simulink model "Model"  (R2018a)
settings: Solver=VariableStepAuto  StartTime=0.0  StopTime=1000  FixedStep=1/480  RelTol=1e-2  EnableMultiTasking=on
model workspace (MAT data in the model file):
  t = Simulink.Parameter
  t.DataType = 'auto'
  t.Dimensions = [0 0]
undefined symbols (not defined in the file or in its folder): deg, Earth, F, Light, MIL, rad, Receive, s, Send, WGS84
libraries: simulink_extras x7, aerolibfltsims x4, aerolibconvert2 x4, aerolibwind2 x3, aerolibtransform2 x1, aerolibatmos2 x1, sharedtransform x1, aerolibanimutils x1, aerolibasang x1
settings Model: Creator=venge  LastModifiedBy=venge
settings SolverCC: AlgebraicLoopSolver=LineSearch  AutoInsertRateTranBlk=on
settings OptimizationCC: LifeSpan=inf
settings DebuggingCC: MaxConsecutiveZCsMsg=warning  ModelReferenceExtraNoncontSigs=warning  SFUnexpectedBacktrackingDiag=warning  SFNoUnconditionalDefaultTransitionDiag=warning  SFExecutionAtInitializationDiag=none
settings CodeAppCC: StateflowObjectComments=on
settings GRTTargetCC: TargetLangStandard=C89/C90 (ANSI)  GeneratePreprocessorConditionals=Disable all
settings ConfigComp: CovMetricSettings=dw  CovHtmlReporting=on  CovSaveCumulativeToWorkspaceVar=on  CovSaveSingleToWorkspaceVar=on  CovExternalEMLEnable=off

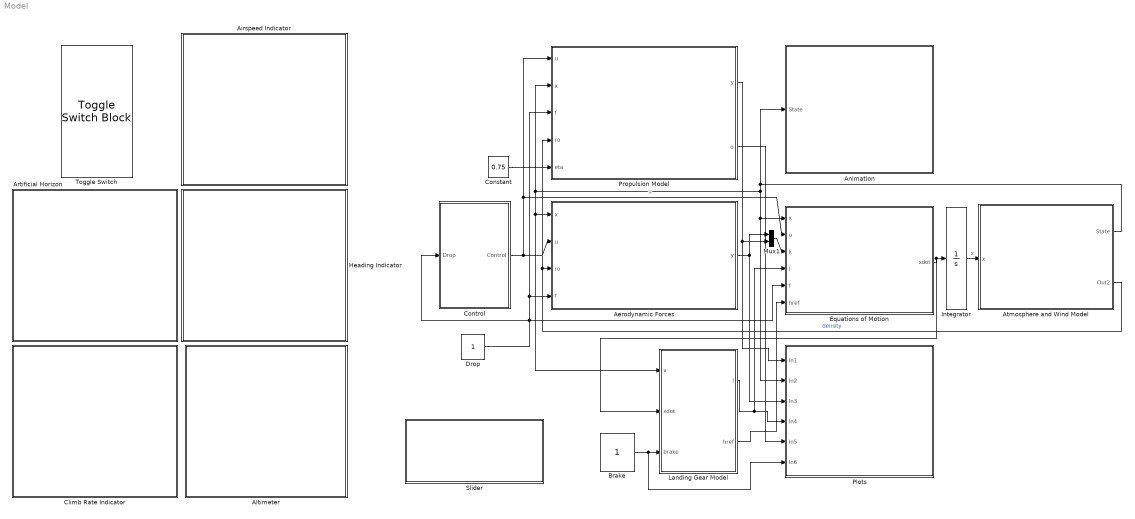
== system Model ==
  "Aerodynamic Forces " : MATLAB Function  TreatAsAtomicUnit=on
  Airspeed Indicator : Subsystem  DialogController=aeroblksHMICreateDDGDialog  IsWebBlock=on  mask(MWDashboardBlock){webBlockId=31f690db-bb0a-4ac4-9dff-202d3d07e85e, webBlockType=airspeedindicator, ShowInLibBrowser=on, ShowInitialText=on, HMISrcModelName=Model}
      mask prompts: webBlockId "WebBlock Id"; webBlockType "WebBlock Type"; HMISrcModelName "Source Model"
      mask help: aeroblksHMI:aeroblkhmi:AirspeedIndicatorDialogDesc
      mask Help: eval('asbhmihelp(''airspeedindicator'')');
      mask Display:
      | if strcmp(get_param(bdroot(gcb),'BlockDiagramType'), 'library')
      |  image([(matlabroot) '/toolbox/aeroblks/aeroblks/hmi/icons/AirspeedIndicatorIcon.svg'])
      | end
  Altimeter : Subsystem  DialogController=aeroblksHMICreateDDGDialog  IsWebBlock=on  mask(MWDashboardBlock){webBlockId=98444758-a21f-440e-aafb-46ae4afdabfa, webBlockType=altimeter, ShowInLibBrowser=on, ShowInitialText=on, HMISrcModelName=Model}
      mask prompts: webBlockId "WebBlock Id"; webBlockType "WebBlock Type"; HMISrcModelName "Source Model"
      mask help: aeroblksHMI:aeroblkhmi:AltimeterDialogDesc
      mask Help: eval('asbhmihelp(''altimeter'')');
      mask Display:
      | if strcmp(get_param(bdroot(gcb),'BlockDiagramType'), 'library')
      |  image([(matlabroot) '/toolbox/aeroblks/aeroblks/hmi/icons/AltimeterIcon.svg'])
      | end
  Animation : Subsystem
      mask Display: image('C:\Users\venge\Documents\Thesis\Flight_Simulator\assets\Animation.png');
  Artificial Horizon : Subsystem  DialogController=aeroblksHMICreateDDGDialog  IsWebBlock=on  mask(MWDashboardBlock){webBlockId=0a6384c6-9f4b-45f8-990f-726f75900e1f, webBlockType=artificialhorizon, ShowInLibBrowser=on, ShowInitialText=on, HMISrcModelName=Model}
      mask prompts: webBlockId "WebBlock Id"; webBlockType "WebBlock Type"; HMISrcModelName "Source Model"
      mask help: aeroblksHMI:aeroblkhmi:ArtificialHorizonDialogDesc
      mask Help: eval('asbhmihelp(''artificialhorizon'')');
      mask Display:
      | if strcmp(get_param(bdroot(gcb),'BlockDiagramType'), 'library')
      |  image([(matlabroot) '/toolbox/aeroblks/aeroblks/hmi/icons/ArtificialHorizonIcon.svg'])
      | end
  Atmosphere and Wind Model : Subsystem
      mask Display: image('C:\Users\venge\Documents\Thesis\Flight_Simulator\assets\Wind.jpg');
  Climb Rate Indicator : Subsystem  DialogController=aeroblksHMICreateDDGDialog  IsWebBlock=on  mask(MWDashboardBlock){webBlockId=41f67cdb-ffed-4f88-bf4d-534dd7e67a65, webBlockType=climbindicator, ShowInLibBrowser=on, ShowInitialText=on, HMISrcModelName=Model}
      mask prompts: webBlockId "WebBlock Id"; webBlockType "WebBlock Type"; HMISrcModelName "Source Model"
      mask help: aeroblksHMI:aeroblkhmi:ClimbIndicatorDialogDesc
      mask Help: eval('asbhmihelp(''climbindicator'')');
      mask Display:
      | if strcmp(get_param(bdroot(gcb),'BlockDiagramType'), 'library')
      |  image([(matlabroot) '/toolbox/aeroblks/aeroblks/hmi/icons/ClimbIndicatorIcon.svg'])
      | end
  Constant : Constant  Value=0.75
  Control : Subsystem
      mask Display: image('C:\Users\venge\Documents\Thesis\Flight_Simulator\assets\Joystick.jpg');
  Drop : Constant
  "Equations of Motion " : MATLAB Function  TreatAsAtomicUnit=on
  Heading Indicator : Subsystem  DialogController=aeroblksHMICreateDDGDialog  IsWebBlock=on  mask(MWDashboardBlock){webBlockId=bb5b7226-34b9-44e0-9042-3ee55364d958, webBlockType=headingindicator, ShowInLibBrowser=on, ShowInitialText=on, HMISrcModelName=Model}
      mask prompts: webBlockId "WebBlock Id"; webBlockType "WebBlock Type"; HMISrcModelName "Source Model"
      mask help: aeroblksHMI:aeroblkhmi:HeadingIndicatorDialogDesc
      mask Help: eval('asbhmihelp(''headingindicator'')');
      mask Display:
      | if strcmp(get_param(bdroot(gcb),'BlockDiagramType'), 'library')
      |  image([(matlabroot) '/toolbox/aeroblks/aeroblks/hmi/icons/HeadingIndicatorIcon.svg'])
      | end
  Integrator : Integrator  InitialCondition=[30 0 0 0 0 0 0 0 0 0 0 -50]'
  Landing Gear Model : Subsystem
      mask Display: image('C:\Users\venge\Documents\Thesis\Flight_Simulator\assets\LandingGear.jpeg');
  Mux1 : Mux  Inputs=2
  Plots : Subsystem
      mask Display: image('C:\Users\venge\Documents\Thesis\Flight_Simulator\assets\Graph.jpg');
  Propulsion Model : MATLAB Function  TreatAsAtomicUnit=on
  Slider : Subsystem  DialogController=hmiCreateDDGDialog  IsWebBlock=on  mask(MWDashboardBlock){webBlockId=e69ca618-8fcc-4738-b870-e52728e9a647, webBlockType=slider, ShowInLibBrowser=on, ShowInitialText=on, HMISrcModelName=Model}
      mask prompts: webBlockId "WebBlock Id"; webBlockType "WebBlock Type"; HMISrcModelName "Source Model"
      mask help: SimulinkHMI:dialogs:SliderDialogDesc
      mask Help: helpview([docroot '/mapfiles/simulink.map'], 'hmi_slider')
      mask Display:
      | if strcmp(get_param(bdroot(gcb),'BlockDiagramType'), 'library')
      |     image([(matlabroot) '/toolbox/simulink/hmi/icons/Slider.png']);
      | end
  Toggle Switch : ToggleSwitchBlock  WebBlockId=379  LabelPosition=Hide
      settings: Values={{'Off', 'On'}, [0 1]}
  Βrake : Constant
  wires:
  Control/1(Control) -> "Equations of Motion "/2(u), Propulsion Model/1(u), "Aerodynamic Forces "/2(u)  "u"
  "Aerodynamic Forces "/1(y) -> Mux1/1, Plots/3(In3)
  Propulsion Model/1(y) -> Plots/1(In1), Mux1/2
  Mux1/1 -> "Equations of Motion "/3(k)
  Atmosphere and Wind Model/1(State) -> Plots/2(In2), "Equations of Motion "/1(x), Propulsion Model/2(x), Landing Gear Model/1(x), "Aerodynamic Forces "/1(x), Animation/1(State)
  Integrator/1 -> Atmosphere and Wind Model/1(x)  "x"
  Landing Gear Model/1(l) -> Plots/4(In4), "Equations of Motion "/4(l)
  Βrake/1 -> Plots/6(In6), Landing Gear Model/3(brake)
  Atmosphere and Wind Model/2(Out2) -> Propulsion Model/4(ro), "Aerodynamic Forces "/3(ro)  "density"
  "Equations of Motion "/1(xdot) -> Landing Gear Model/2(xdot), Integrator/1
  Drop/1 -> Control/1(Drop), Propulsion Model/3(f), "Aerodynamic Forces "/4(f), "Equations of Motion "/5(f)
  Propulsion Model/2(o) -> Plots/5(In5)
  Constant/1 -> Propulsion Model/5(eta)
  Landing Gear Model/2(href) -> "Equations of Motion "/6(href)

== system Model/Airspeed Indicator ==

== system Model/Altimeter ==

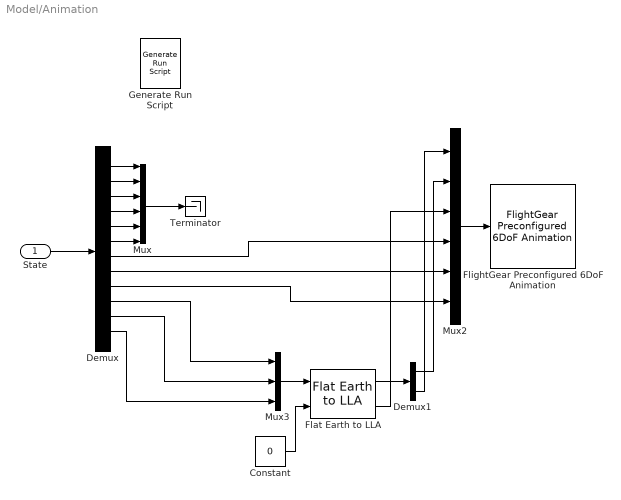
== system Model/Animation ==
  State : Inport
  Constant : Constant  Value=0
  Demux : Demux  Outputs=12
  Demux1 : Demux  Outputs=2
  Flat Earth to LLA : aerolibtransform2/Flat Earth to LLA  units=Metric (MKS)  ptype=Earth (WGS84)  F=1/298.257223563  R=6378137  LL0=[37.6069 -122.381]  psi=0
  FlightGear Preconfigured 6DoF Animation : aerolibfltsims/FlightGear Preconfigured 6DoF Animation  xFlightGearVersion=v2017.3  DestinationIpAddress=127.0.0.1  DestinationPort=5502  SampleTime=1/30
      settings: SourceProductName=Aerospace Blockset
  Generate Run Script : aerolibfltsims/Generate Run Script  Architecture=Default  dataFlow=Send-Receive  GeometryModelName=c172p  AirportId=KSFO  RunwayId=10L  InitialAltitude=2000  InitialHeading=0  OffsetDistance=0  OffsetAzimuth=0  InstallScenery=on  DisableShaders=on  OriginAddress=127.0.0.1  DestinationPort=5502  OriginPort=5505  LocalAddress=127.0.0.1  OutputFileName=runfg_send_recieve.bat  FlightGearBaseDirectory=C:\Program Files\FlightGear 2017.3.1
  Mux : Mux  Inputs=6
  Mux2 : Mux  Inputs=6
  Mux3 : Mux  Inputs=3
  Terminator : Terminator
  wires:
  Demux1/2 -> Mux2/1
  Flat Earth to LLA/1 -> Demux1/1
  Demux1/1 -> Mux2/2
  Mux2/1 -> FlightGear Preconfigured 6DoF Animation/1
  Flat Earth to LLA/2 -> Mux2/3
  Mux3/1 -> Flat Earth to LLA/1
  State/1 -> Demux/1
  Demux/10 -> Mux3/1
  Demux/11 -> Mux3/2
  Demux/12 -> Mux3/3
  Demux/7 -> Mux2/4
  Demux/9 -> Mux2/6
  Demux/6 -> Mux/6
  Demux/5 -> Mux/5
  Demux/4 -> Mux/4
  Demux/3 -> Mux/3
  Demux/2 -> Mux/2
  Demux/1 -> Mux/1
  Mux/1 -> Terminator/1
  Demux/8 -> Mux2/5
  Constant/1 -> Flat Earth to LLA/2

== system Model/Artificial Horizon ==

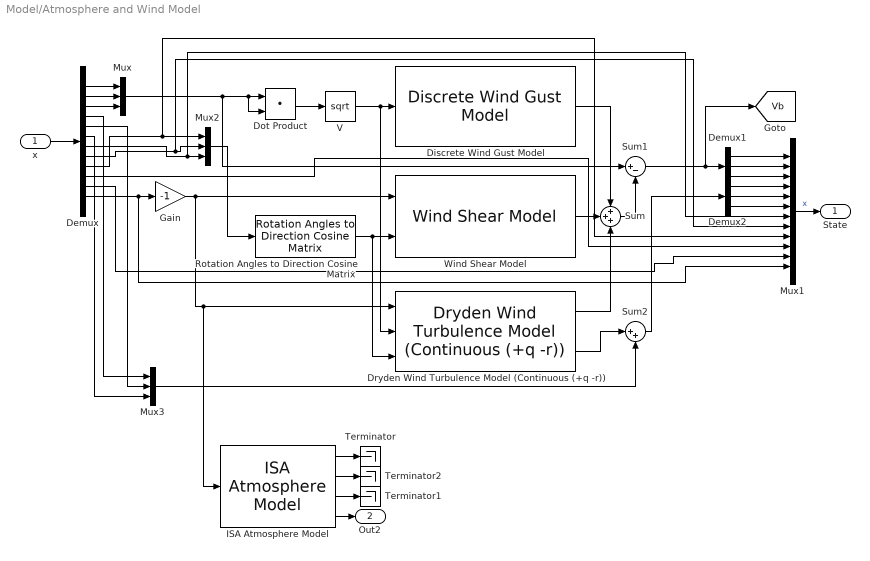
== system Model/Atmosphere and Wind Model ==
  x : Inport
  Demux : Demux  Outputs=12
  Demux1 : Demux  Outputs=3
  Demux2 : Demux  Outputs=3
  Discrete Wind Gust Model : aerolibwind2/Discrete Wind Gust Model  units=Metric (MKS)  Gx=off  Gy=off  Gz=off  t_0=50  d_m=[200 200 200]  v_m=[20 -20 20]
      settings: SourceProductName=Aerospace Blockset
  Dot Product : DotProduct  InputSameDT=on  OutDataTypeStr=Inherit: Inherit via internal rule
  Dryden Wind Turbulence Model (Continuous (+q -r)) : aerolibwind2/Dryden Wind Turbulence Model  (Continuous (+q -r))  units=Metric (MKS)  spec=MIL-F-8785C  model=Continuous Dryden (-q +r)  W20=0  Wdeg=0  TurbProb=10^-2 - Light  L_high=533.4  Wingspan=7.146  ts=0.1  Seed=[23341 23342 23343 23344]  T_on=off
      settings: SourceProductName=Aerospace Blockset
  Gain : Gain  Gain=-1
  ISA Atmosphere Model : aerolibatmos2/ISA Atmosphere Model  custom=off  g=9.80665  gamma=1.4  R=287.0531  L=0.0065  h_trop=11000  h_strat=20000  rho0=1.225  P0=101325  T0=288.15  h0=0
      settings: SourceProductName=Aerospace Blockset
  Mux : Mux  Inputs=3
  Mux1 : Mux  Inputs=12
  Mux2 : Mux  Inputs=3
  Mux3 : Mux  Inputs=3
  Rotation Angles to Direction Cosine Matrix : sharedtransform/Rotation Angles to Direction Cosine Matrix  rotationOrder=ZYX  aMode=aMode
      settings: SourceProductBaseCode=AE
  Sum : Sum  Inputs=+++
  Sum1 : Sum  Inputs=|+-
  Sum2 : Sum  Inputs=|++
  Terminator : Terminator
  Terminator1 : Terminator
  Terminator2 : Terminator
  V : Sqrt  SaturateOnIntegerOverflow=on
  Wind Shear Model : aerolibwind2/Wind Shear Model  units=Metric (MKS)  phase=Other  W_20=0  Wdeg=0
      settings: SourceProductName=Aerospace Blockset
  State : Outport  PortDimensions=12
  Out2 : Outport  Port=2
  tag scope: Vb=global
  wires:
  Demux/2 -> Mux/2
  Demux/3 -> Mux/3
  Demux/1 -> Mux/1
  Sum2/1 -> Demux2/1
  Mux3/1 -> Sum2/2
  Mux/1 -> Sum1/1, Dot Product/2, Dot Product/1
  Mux2/1 -> Rotation Angles to Direction Cosine Matrix/1
  Gain/1 -> ISA Atmosphere Model/1, Dryden Wind Turbulence Model (Continuous (+q -r))/1, Wind Shear Model/1
  Demux/12 -> Mux1/12, Gain/1
  Discrete Wind Gust Model/1 -> Sum/1
  Sum/1 -> Sum1/2
  V/1 -> Dryden Wind Turbulence Model (Continuous (+q -r))/2, Discrete Wind Gust Model/1
  Rotation Angles to Direction Cosine Matrix/1 -> Dryden Wind Turbulence Model (Continuous (+q -r))/3, Wind Shear Model/2
  Dryden Wind Turbulence Model (Continuous (+q -r))/1 -> Sum/3
  Dot Product/1 -> V/1
  Wind Shear Model/1 -> Sum/2
  Dryden Wind Turbulence Model (Continuous (+q -r))/2 -> Sum2/1
  Mux1/1 -> State/1  "x"
  x/1 -> Demux/1
  Demux1/1 -> Mux1/1
  Demux1/2 -> Mux1/2
  Demux1/3 -> Mux1/3
  Demux/4 -> Mux3/1
  Demux/5 -> Mux3/2
  Demux/6 -> Mux3/3
  Demux/7 -> Mux1/7, Mux2/3
  Demux/8 -> Mux1/8, Mux2/2
  Demux/9 -> Mux1/9, Mux2/1
  Demux/10 -> Mux1/10
  Demux/11 -> Mux1/11
  Demux2/1 -> Mux1/4
  Demux2/2 -> Mux1/5
  Demux2/3 -> Mux1/6
  ISA Atmosphere Model/3 -> Terminator1/1
  ISA Atmosphere Model/1 -> Terminator/1
  ISA Atmosphere Model/2 -> Terminator2/1
  ISA Atmosphere Model/4 -> Out2/1
  Sum1/1 -> [Vb], Demux1/1

== system Model/Climb Rate Indicator ==

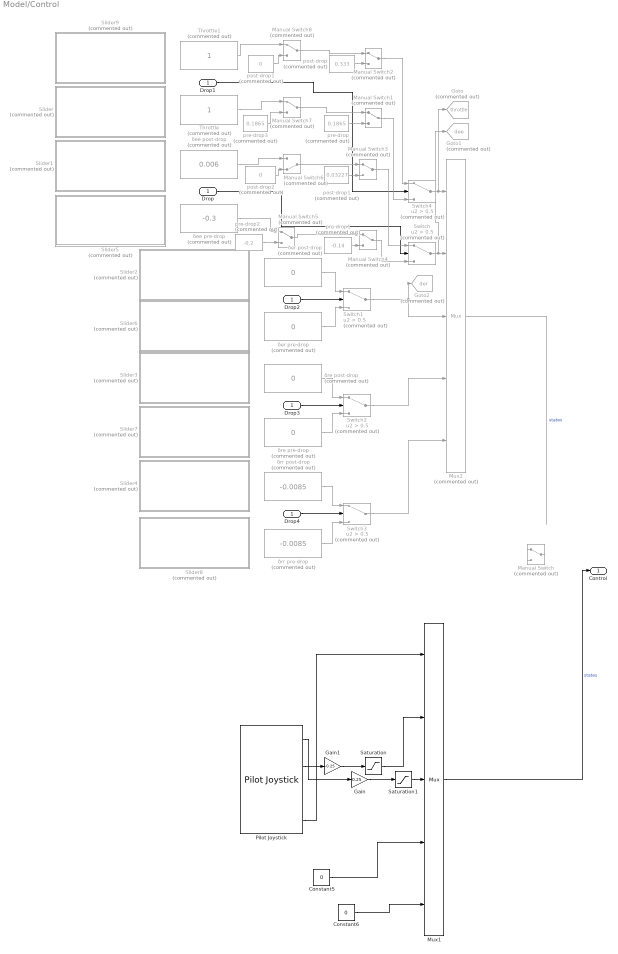
== system Model/Control ==
  Drop : Inport
  Constant5 : Constant  Value=0
  Constant6 : Constant  Value=0
  Drop{1..4} (4 alike) : InportShadow
  Gain : Gain  Gain=0.25
  Gain1 : Gain  Gain=-0.25
  Goto : Goto  Commented=on  GotoTag=throttle  TagVisibility=global
  Goto1 : Goto  Commented=on  GotoTag=dee  TagVisibility=global
  Goto2 : Goto  Commented=on  GotoTag=der  TagVisibility=global
  Manual Switch{,1..5,7..8} (8 alike) : ManualSwitch  Commented=on
  Manual Switch6 : ManualSwitch  Commented=on  CurrentSetting=0
  Mux1 : Mux  Inputs=5
  Mux2 : Mux  Commented=on  Inputs=5
  Pilot Joystick : aerolibanimutils/Pilot Joystick  JoystickID=Joystick1  OutputConfiguration=FourAxis  SampleTime=1/30
  Saturation : Saturate  UpperLimit=0.4  LowerLimit=-0.4
  Saturation1 : Saturate  UpperLimit=0.4  LowerLimit=-0.4
  Slider : Subsystem  Commented=on  DialogController=hmiCreateDDGDialog  IsWebBlock=on  mask(MWDashboardBlock){webBlockId=71ff8332-cc57-48c6-a6db-909c0a3f45d7, webBlockType=slider, ShowInLibBrowser=on, ShowInitialText=on, HMISrcModelName=Model}
      mask prompts: webBlockId "WebBlock Id"; webBlockType "WebBlock Type"; HMISrcModelName "Source Model"
      mask Help: helpview([docroot '/mapfiles/simulink.map'], 'hmi_slider')
      mask Display:
      | if strcmp(get_param(bdroot(gcb),'BlockDiagramType'), 'library')
      |     image([(matlabroot) '/toolbox/simulink/hmi/icons/Slider.png']);
      | end
  Slider1 : Subsystem  Commented=on  DialogController=hmiCreateDDGDialog  IsWebBlock=on  mask(MWDashboardBlock){webBlockId=76778588-3397-48c9-bd33-f2999619dd82, webBlockType=slider, ShowInLibBrowser=on, ShowInitialText=on, HMISrcModelName=Model}
      mask prompts: webBlockId "WebBlock Id"; webBlockType "WebBlock Type"; HMISrcModelName "Source Model"
      mask Help: helpview([docroot '/mapfiles/simulink.map'], 'hmi_slider')
      mask Display:
      | if strcmp(get_param(bdroot(gcb),'BlockDiagramType'), 'library')
      |     image([(matlabroot) '/toolbox/simulink/hmi/icons/Slider.png']);
      | end
  Slider2 : Subsystem  Commented=on  DialogController=hmiCreateDDGDialog  IsWebBlock=on  mask(MWDashboardBlock){webBlockId=50b965dc-06ed-4b8f-b83d-27d9610c145d, webBlockType=slider, ShowInLibBrowser=on, ShowInitialText=on, HMISrcModelName=Model}
      mask prompts: webBlockId "WebBlock Id"; webBlockType "WebBlock Type"; HMISrcModelName "Source Model"
      mask Help: helpview([docroot '/mapfiles/simulink.map'], 'hmi_slider')
      mask Display:
      | if strcmp(get_param(bdroot(gcb),'BlockDiagramType'), 'library')
      |     image([(matlabroot) '/toolbox/simulink/hmi/icons/Slider.png']);
      | end
  Slider3 : Subsystem  Commented=on  DialogController=hmiCreateDDGDialog  IsWebBlock=on  mask(MWDashboardBlock){webBlockId=b80eeb05-1d01-4bba-9885-77def870bdbb, webBlockType=slider, ShowInLibBrowser=on, ShowInitialText=on, HMISrcModelName=Model}
      mask prompts: webBlockId "WebBlock Id"; webBlockType "WebBlock Type"; HMISrcModelName "Source Model"
      mask Help: helpview([docroot '/mapfiles/simulink.map'], 'hmi_slider')
      mask Display:
      | if strcmp(get_param(bdroot(gcb),'BlockDiagramType'), 'library')
      |     image([(matlabroot) '/toolbox/simulink/hmi/icons/Slider.png']);
      | end
  Slider4 : Subsystem  Commented=on  DialogController=hmiCreateDDGDialog  IsWebBlock=on  mask(MWDashboardBlock){webBlockId=fbe885e3-15c5-4246-8884-16500feaa139, webBlockType=slider, ShowInLibBrowser=on, ShowInitialText=on, HMISrcModelName=Model}
      mask prompts: webBlockId "WebBlock Id"; webBlockType "WebBlock Type"; HMISrcModelName "Source Model"
      mask Help: helpview([docroot '/mapfiles/simulink.map'], 'hmi_slider')
      mask Display:
      | if strcmp(get_param(bdroot(gcb),'BlockDiagramType'), 'library')
      |     image([(matlabroot) '/toolbox/simulink/hmi/icons/Slider.png']);
      | end
  Slider5 : Subsystem  Commented=on  DialogController=hmiCreateDDGDialog  IsWebBlock=on  mask(MWDashboardBlock){webBlockId=8ae96144-d421-4708-bdd7-b0b2312d1c18, webBlockType=slider, ShowInLibBrowser=on, ShowInitialText=on, HMISrcModelName=Model}
      mask prompts: webBlockId "WebBlock Id"; webBlockType "WebBlock Type"; HMISrcModelName "Source Model"
      mask Help: helpview([docroot '/mapfiles/simulink.map'], 'hmi_slider')
      mask Display:
      | if strcmp(get_param(bdroot(gcb),'BlockDiagramType'), 'library')
      |     image([(matlabroot) '/toolbox/simulink/hmi/icons/Slider.png']);
      | end
  Slider6 : Subsystem  Commented=on  DialogController=hmiCreateDDGDialog  IsWebBlock=on  mask(MWDashboardBlock){webBlockId=9b86d56f-dae5-440b-8eb5-941c5f267d11, webBlockType=slider, ShowInLibBrowser=on, ShowInitialText=on, HMISrcModelName=Model}
      mask prompts: webBlockId "WebBlock Id"; webBlockType "WebBlock Type"; HMISrcModelName "Source Model"
      mask Help: helpview([docroot '/mapfiles/simulink.map'], 'hmi_slider')
      mask Display:
      | if strcmp(get_param(bdroot(gcb),'BlockDiagramType'), 'library')
      |     image([(matlabroot) '/toolbox/simulink/hmi/icons/Slider.png']);
      | end
  Slider7 : Subsystem  Commented=on  DialogController=hmiCreateDDGDialog  IsWebBlock=on  mask(MWDashboardBlock){webBlockId=463fa428-adca-439c-b2e0-0a9da63c573c, webBlockType=slider, ShowInLibBrowser=on, ShowInitialText=on, HMISrcModelName=Model}
      mask prompts: webBlockId "WebBlock Id"; webBlockType "WebBlock Type"; HMISrcModelName "Source Model"
      mask Help: helpview([docroot '/mapfiles/simulink.map'], 'hmi_slider')
      mask Display:
      | if strcmp(get_param(bdroot(gcb),'BlockDiagramType'), 'library')
      |     image([(matlabroot) '/toolbox/simulink/hmi/icons/Slider.png']);
      | end
  Slider8 : Subsystem  Commented=on  DialogController=hmiCreateDDGDialog  IsWebBlock=on  mask(MWDashboardBlock){webBlockId=151de3c8-e2fa-4a35-b614-725181a5af33, webBlockType=slider, ShowInLibBrowser=on, ShowInitialText=on, HMISrcModelName=Model}
      mask prompts: webBlockId "WebBlock Id"; webBlockType "WebBlock Type"; HMISrcModelName "Source Model"
      mask Help: helpview([docroot '/mapfiles/simulink.map'], 'hmi_slider')
      mask Display:
      | if strcmp(get_param(bdroot(gcb),'BlockDiagramType'), 'library')
      |     image([(matlabroot) '/toolbox/simulink/hmi/icons/Slider.png']);
      | end
  Slider9 : Subsystem  Commented=on  DialogController=hmiCreateDDGDialog  IsWebBlock=on  mask(MWDashboardBlock){webBlockId=f535e40a-6bfd-4d60-87e7-b92c922fa0f7, webBlockType=slider, ShowInLibBrowser=on, ShowInitialText=on, HMISrcModelName=Model}
      mask prompts: webBlockId "WebBlock Id"; webBlockType "WebBlock Type"; HMISrcModelName "Source Model"
      mask Help: helpview([docroot '/mapfiles/simulink.map'], 'hmi_slider')
      mask Display:
      | if strcmp(get_param(bdroot(gcb),'BlockDiagramType'), 'library')
      |     image([(matlabroot) '/toolbox/simulink/hmi/icons/Slider.png']);
      | end
  Switch{,1..4} (5 alike) : Switch  Commented=on  Criteria=u2 > Threshold  Threshold=0.5
  Throttle : Constant  Commented=on
  Throttle1 : Constant  Commented=on
  post-drop1 : Constant  Commented=on  Value=0.03227
  post-drop2 : Constant  Commented=on  Value=0
  pre-drop : Constant  Commented=on  Value=0.1865
  pre-drop1 : Constant  Commented=on  Value=-0.14
  pre-drop2 : Constant  Commented=on  Value=-0.2
  pre-drop3 : Constant  Commented=on  Value=0.1865
  pοst-drop : Constant  Commented=on  Value=0.333
  pοst-drop1 : Constant  Commented=on  Value=0
  δee post-drop : Constant  Commented=on  Value=0.006
  δee pre-drop : Constant  Commented=on  Value=-0.3
  δer post-drop : Constant  Commented=on  Value=0
  δer pre-drop : Constant  Commented=on  Value=0
  δre post-drop : Constant  Commented=on  Value=0
  δre pre-drop : Constant  Commented=on  Value=0
  δrr post-drop : Constant  Commented=on  Value=-0.0085
  δrr pre-drop : Constant  Commented=on  Value=-0.0085
  Control : Outport
  wires:
  Mux1/1 -> Control/1  "states"
  Pilot Joystick/4 -> Mux1/1
  Pilot Joystick/1 -> Gain/1
  Pilot Joystick/2 -> Gain1/1
  δrr post-drop/1 -> Switch3/1
  δer post-drop/1 -> Switch1/1
  Gain1/1 -> Saturation/1
  Constant5/1 -> Mux1/4
  Gain/1 -> Saturation1/1
  Constant6/1 -> Mux1/5
  Saturation/1 -> Mux1/2
  Saturation1/1 -> Mux1/3
  Switch/1 -> Goto1/1, Mux2/2
  Switch1/1 -> Goto2/1, Mux2/3
  Switch2/1 -> Mux2/4
  Switch3/1 -> Mux2/5
  δee post-drop/1 -> Manual Switch6/1
  δre post-drop/1 -> Switch2/1
  δer pre-drop/1 -> Switch1/3
  δrr pre-drop/1 -> Switch3/3
  δre pre-drop/1 -> Switch2/3
  Mux2/1 -> ?  "states"
  Drop/1 -> Switch/2
  Drop4/1 -> Switch3/2
  Drop3/1 -> Switch2/2
  Drop2/1 -> Switch1/2
  Throttle/1 -> Manual Switch7/1
  δee pre-drop/1 -> Manual Switch5/1
  Switch4/1 -> Goto/1, Mux2/1
  Drop1/1 -> Switch4/2
  Throttle1/1 -> Manual Switch8/1
  pre-drop/1 -> Manual Switch1/2
  Manual Switch1/1 -> Switch4/3
  pοst-drop/1 -> Manual Switch2/2
  Manual Switch2/1 -> Switch4/1
  Manual Switch3/1 -> Switch/1
  post-drop1/1 -> Manual Switch3/2
  Manual Switch4/1 -> Switch/3
  pre-drop1/1 -> Manual Switch4/2
  Manual Switch5/1 -> Manual Switch4/1
  pre-drop2/1 -> Manual Switch5/2
  Manual Switch6/1 -> Manual Switch3/1
  post-drop2/1 -> Manual Switch6/2
  Manual Switch7/1 -> Manual Switch1/1
  Manual Switch8/1 -> Manual Switch2/1
  pοst-drop1/1 -> Manual Switch8/2
  pre-drop3/1 -> Manual Switch7/2

== system Model/Heading Indicator ==

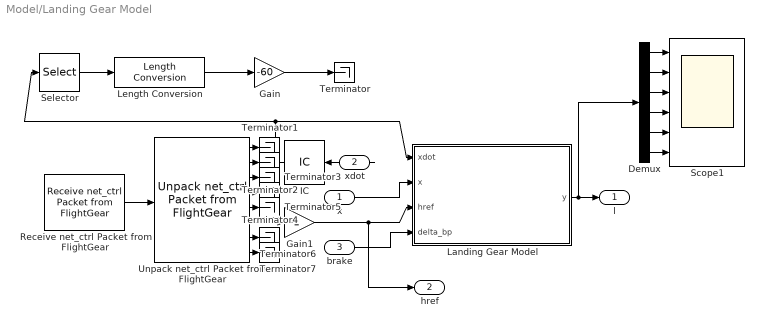
== system Model/Landing Gear Model ==
  x : Inport
  xdot : Inport  Port=2
  brake : Inport  Port=3
  Demux : Demux  Outputs=6
  Gain : Gain  Gain=-60
  Gain1 : Gain  Gain=-1
  IC : InitialCondition  Value=[0 0 0 0 0 0 0 0 0 0 0 0]'
  Landing Gear Model : MATLAB Function  TreatAsAtomicUnit=on
  Length Conversion : aerolibconvert2/Length Conversion  IU=m  OU=ft
  Receive net_ctrl Packet from FlightGear : aerolibfltsims/Receive net_ctrl Packet from FlightGear  FlightGearVersion=v2017.3  ReceiveAddress=127.0.0.1  ReceivePort=5505  ReceiveWidth=744  varLen=off  SampleTime=1/30  packetFlag=off
      settings: AttributesFormatString=Version Selected:\n%<FlightGearVersion>  SourceProductName=Aerospace Blockset  SourceProductBaseCode=AE
  Scope1 : Scope  NumInputPorts=6
  Selector : Selector  InputPortWidth=12  IndexOptions=Index vector (dialog)  Indices=[12]  OutputSizes=1
  Terminator{,1..7} (8 alike) : Terminator
  Unpack net_ctrl Packet from FlightGear : aerolibfltsims/Unpack net_ctrl Packet from FlightGear  FlightGearVersion=v2017.3  ShowControlSurfacePositionOutputs=off  ShowEngineFuelOutputs=off  ShowLandingGearOutputs=off  ShowAvionicOutputs=off  ShowEnvironmentOutputs=on  SampleTime=1/30
      settings: AttributesFormatString=Version Selected: %<FlightGearVersion>  SourceProductName=Aerospace Blockset  SourceProductBaseCode=AE
  l : Outport
  href : Outport  Port=2
  wires:
  IC/1 -> Selector/1, Landing Gear Model/1(xdot)
  Landing Gear Model/1(y) -> Demux/1, l/1
  x/1 -> Landing Gear Model/2(x)
  xdot/1 -> IC/1
  brake/1 -> Landing Gear Model/4(delta_bp)
  Selector/1 -> Length Conversion/1
  Gain/1 -> Terminator/1
  Length Conversion/1 -> Gain/1
  Unpack net_ctrl Packet from FlightGear/6 -> Gain1/1
  Gain1/1 -> href/1, Landing Gear Model/3(href)
  Receive net_ctrl Packet from FlightGear/1 -> Unpack net_ctrl Packet from FlightGear/1
  Demux/1 -> Scope1/1
  Demux/2 -> Scope1/2
  Demux/3 -> Scope1/3
  Demux/4 -> Scope1/4
  Demux/5 -> Scope1/5
  Demux/6 -> Scope1/6
  Unpack net_ctrl Packet from FlightGear/1 -> Terminator1/1
  Unpack net_ctrl Packet from FlightGear/2 -> Terminator2/1
  Unpack net_ctrl Packet from FlightGear/3 -> Terminator3/1
  Unpack net_ctrl Packet from FlightGear/4 -> Terminator4/1
  Unpack net_ctrl Packet from FlightGear/5 -> Terminator5/1
  Unpack net_ctrl Packet from FlightGear/7 -> Terminator6/1
  Unpack net_ctrl Packet from FlightGear/8 -> Terminator7/1

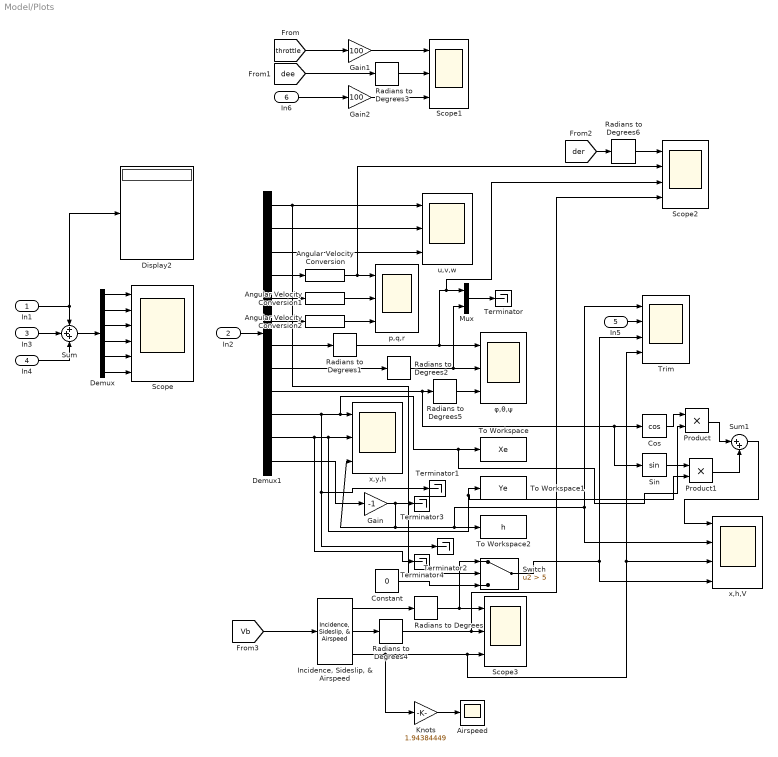
== system Model/Plots ==
  In1 : Inport
  In2 : Inport  Port=2
  In3 : Inport  Port=3
  In4 : Inport  Port=4
  In5 : Inport  Port=5
  In6 : Inport  Port=6
  Airspeed : Scope
  Angular Velocity Conversion : aerolibconvert2/Angular Velocity Conversion  IU=rad/s  OU=deg/s
      settings: SourceProductName=Aerospace Blockset
  Angular Velocity Conversion1 : aerolibconvert2/Angular Velocity Conversion  IU=rad/s  OU=deg/s
      settings: SourceProductName=Aerospace Blockset
  Angular Velocity Conversion2 : aerolibconvert2/Angular Velocity Conversion  IU=rad/s  OU=deg/s
      settings: SourceProductName=Aerospace Blockset
  Constant : Constant  Value=0
  Cos : Trigonometry  Operator=cos
  Demux : Demux  Outputs=6
  Demux1 : Demux  Outputs=12
  Display2 : Display
  Gain : Gain  Gain=-1
  Gain1 : Gain  Gain=100
  Gain2 : Gain  Gain=100
  "Incidence, Sideslip, & Airspeed" : aerolibasang/Incidence, Sideslip, & Airspeed
      settings: SourceProductName=Aerospace Blockset
  Knots : Gain  Gain=1.94384449
  Mux : Mux  Inputs=2
  Product : Product
  Product1 : Product
  Radians to Degrees{,1..6} (7 alike) : simulink_extras/Transformations/Radians to Degrees
  Scope : Scope  NumInputPorts=6
  Scope1 : Scope  NumInputPorts=3
  Scope2 : Scope  NumInputPorts=4
  Scope3 : Scope  NumInputPorts=3
  Sin : Trigonometry
  Sum : Sum  Inputs=+++
  Sum1 : Sum  Inputs=|++
  Switch : Switch  Criteria=u2 > Threshold  Threshold=5
  Terminator{,1..4} (5 alike) : Terminator
  To Workspace : ToWorkspace  VariableName=Xe  SampleTime=-1
  To Workspace1 : ToWorkspace  VariableName=Ye  SampleTime=-1
  To Workspace2 : ToWorkspace  VariableName=h  SampleTime=-1
  Trim : Scope  NumInputPorts=4
  p,q,r : Scope  NumInputPorts=3
  u,v,w : Scope  NumInputPorts=3
  x,h,V : Scope  NumInputPorts=4
  x,y,h : Scope  NumInputPorts=3
  φ,θ,ψ : Scope  NumInputPorts=3
  wires:
  Demux/4 -> Scope/4
  Demux/6 -> Scope/6
  Demux/5 -> Scope/5
  Sum/1 -> Demux/1
  Demux/3 -> Scope/3
  Demux/2 -> Scope/2
  Demux/1 -> Scope/1
  In4/1 -> Sum/3
  In3/1 -> Sum/2
  In2/1 -> Demux1/1
  Demux1/5 -> Angular Velocity Conversion1/1
  Demux1/9 -> Sin/1, Cos/1, Radians to Degrees5/1
  Radians to Degrees2/1 -> φ,θ,ψ/2, Mux/2
  Radians to Degrees1/1 -> Scope2/3, Mux/1, φ,θ,ψ/1
  Mux/1 -> Terminator/1
  Demux1/1 -> Switch/2, u,v,w/1
  Demux1/6 -> Angular Velocity Conversion2/1
  Demux1/8 -> Radians to Degrees2/1
  Demux1/2 -> u,v,w/2
  Radians to Degrees5/1 -> φ,θ,ψ/3
  Demux1/11 -> Terminator4/1, x,y,h/2, Product1/2, To Workspace1/1
  Demux1/7 -> Radians to Degrees1/1
  Demux1/4 -> Angular Velocity Conversion/1
  Demux1/10 -> Product/2, To Workspace/1, x,y,h/1, Terminator1/1, Terminator2/1
  Demux1/12 -> Gain/1
  Gain/1 -> Terminator3/1, x,y,h/3, x,h,V/2, Trim/1, To Workspace2/1
  Demux1/3 -> u,v,w/3
  Angular Velocity Conversion/1 -> Scope2/2, p,q,r/1
  Angular Velocity Conversion1/1 -> p,q,r/2
  Angular Velocity Conversion2/1 -> p,q,r/3
  [throttle] -> Gain1/1
  Gain1/1 -> Scope1/1
  [dee] -> Radians to Degrees3/1
  Radians to Degrees3/1 -> Scope1/2
  In1/1 -> Display2/1, Sum/1
  Radians to Degrees4/1 -> Scope2/4, Scope3/2
  [Vb] -> "Incidence, Sideslip, & Airspeed"/1
  "Incidence, Sideslip, & Airspeed"/1 -> Radians to Degrees/1
  "Incidence, Sideslip, & Airspeed"/3 -> Trim/4, x,h,V/3, Scope3/3, Knots/1
  "Incidence, Sideslip, & Airspeed"/2 -> Radians to Degrees4/1
  Knots/1 -> Airspeed/1
  In5/1 -> Trim/2
  [der] -> Radians to Degrees6/1
  Radians to Degrees6/1 -> Scope2/1
  In6/1 -> Gain2/1
  Gain2/1 -> Scope1/3
  Radians to Degrees/1 -> Switch/1, Scope3/1
  Constant/1 -> Switch/3
  Switch/1 -> Trim/3, x,h,V/4
  Cos/1 -> Product/1
  Sin/1 -> Product1/1
  Product/1 -> Sum1/1
  Product1/1 -> Sum1/2
  Sum1/1 -> x,h,V/1

== system Model/Slider ==

== system Model/Control/Slider ==

== system Model/Control/Slider1 ==

== system Model/Control/Slider2 ==

== system Model/Control/Slider3 ==

== system Model/Control/Slider4 ==

== system Model/Control/Slider5 ==

== system Model/Control/Slider6 ==

== system Model/Control/Slider7 ==

== system Model/Control/Slider8 ==

== system Model/Control/Slider9 ==

== matlab function Model/Aerodynamic Forces  ==
  data: x input; y output; u input; ro input; f input
function y  = Aerodynamics(x, u, ro, f)
  
  % Aircraft Design Data
  p = struct('sos', 332.4, 'c', 1.005, 'S', 5.306, 'b', 7.146,...
      'Cmref', -0.03, 'Cdref', 0.0222, 'CLref', 0.3617, 'Cy_phat', 0,...
      'phatref', 0, 'Cy_rhat', 0.175, 'rhatref', 0, 'Cy_bhta', -0.513,...
      'bhtaref', 0, 'Cl_bhta', -0.1122, 'Cl_phat', -0.6421,...
      'Cl_rhat', 0.1526, 'CL_qhat', [7.2382 5.8815], 'qhatref', 0,...
      'Cm_qhat', -5.9134, 'Cm_qhat2', -5.3559, 'Cn_bhta', 0.0716,...
      'Cn_phat', 0.0498, 'Cn_phat2', 0.0484, 'Cn_rhat', -0.0524,...
      'stall', 0.2443);
        
  V = velocity(x);  % Velocity
  a = aoa(x);  % Angle of attack
  b = bhta(x);  % Sideslip angle
  deltaee = u(2);  % Elevon as elevator deflection
  deltare = u(4);  % Elevon as rudder deflection
  
  L = 1 / 2 * ro * V .^ 2 * CL(p, x, u, f) * p.S;  % Lift force
  D = 1 / 2 * ro * V .^ 2 * Cd(p, x, u) * p.S;  % Drag force
  Y = 1 / 2 * ro * V .^ 2 * Cy(p, x, u) * p.S;  % Side force
  Lmoment = 1 / 2 * ro * V .^ 2 * p.S * p.b * C_l(p, x, u);  % Rolling moment
  Mmoment = 1 / 2 * ro * V .^ 2 * p.S * p.c * Cm(p, x, u, f);  % Pitching moment
  Nmoment = 1 / 2 * ro * V .^ 2 * p.S * p.b * Cn(p, x, u, f);  % Yawing moment
 
  % Transformation Matrix
  TM = [cos(a) * cos(b), -cos(a) * sin(b), -sin(a);...
        0, 1, 0; sin(a)*cos(b), -sin(a) * sin(b), cos(a)];
 
  % Lift and Drag corrections
  Zcs = 1/2 * ro * V .^ 2 * p.S * (CL_deltaee(deltaee)...
      + CL_deltare(deltare));
  Xcs = 1/2 * ro * V .^ 2 * p.S * (Cd_deltaee(deltaee)...
      + Cd_deltare(deltare));
 
  z = TM * [-(D + Xcs), Y, -(L + Zcs)]'; % Forces translation to earth axes
  
  y = [z(1), z(2), z(3), Lmoment, 1.1 * Mmoment, Nmoment]';
 
end

== matlab function Model/Propulsion Model ==
  data: y output; u input; x input; o output; f input; ro input; eta input
function [y, o] = thrust(u, x, f, ro, eta)

  xcg1 = - 1.897;  % gravity center in x-axis pre-drop
  xcg2 = - 1.9805;  % gravity center in x-axis post-drop
  xT = 2.968;  % thrust origin position in x-axis
  zT = -0.096;  % thrust origin position in z-axis
  eT = 0.03491;  % thrust angle
  
  V = velocity(x);  % aircraft velocity
  P = 177.23 * u(1)^4 - 336.73 * u(1)^3 + 141.73 * u(1)^2 + 60.244 * u(1)...
      - 0.2344;  % engine power
  T = ro/1.225 * 1000 * P * eta / V;  % engine thrust value
  Tx = T * cos(eT);  % x-axis thrust
  Ty = 0;  % y-axis thrust
  Tz = T * sin(eT);  % z-axis thrust
  LT = 0;  % rolling moment due to thrust
  NT = 0;  % yawing moment due to thrust
  % Pitching moment due to thrust
  if f == 0  % pre-drop
      MT = (xT + xcg1) * Tz + zT * Tx;
  else  % post-drop
      MT = (xT + xcg2) * Tz + zT * Tx;
  end
  
  y = [Tx, Ty, Tz, LT, MT, NT]';
  o = T;  % graph output
  
end

== matlab function Model/Equations of Motion  ==
  data: x input; u input; xdot output; k input; l input; f input; href input
function xdot  = EoM(x, u, k, l, f, href)
  
  % Aircraft Design Data
  p = struct('m1', 246.3, 'm2', 187.4357143,'xcg1', 1.897, 'xcg2', 1.9805,...
      'Ixx1', 286.8744056, 'Ixx2', 286.8255, 'Ixy', 0, 'Ixz', 3.208324808,...
      'Iyy1', 134.2579124, 'Iyy2', 126.5266, 'Iyz', 0, 'Izz1', 403.8622993,...
      'Izz2', 396.1506, 'g', 9.81);
  theta = x(8);
  phi = x(7);
  psi = x(9);
  
  if f == 0  % Pre-Drop Conditions
    m = p.m1;  % Mass value
    IB = [p.Ixx1, 0, -p.Ixz; 0, p.Iyy1, 0; -p.Ixz, 0, p.Izz1];  % Inertia Matrix
  else  % Post-drop Conditions
    m = p.m2;  % Mass value
    IB = [p.Ixx2, 0, -p.Ixz; 0, p.Iyy2, 0; -p.Ixz, 0, p.Izz2];  % Inertia Matrix    
  end
  
  mdot = 0;  % Mass variation with time
  IBdot =[0, 0, 0; 0, 0, 0; 0, 0, 0];  % Inertia Matrix variation with time
  
  % Cos - sin Matrix
  B = [cos(theta) * cos(psi), cos(theta) * sin(psi), -sin(theta);...
       -cos(phi) * sin(psi) + sin(phi) * sin(theta) * cos(psi),...
       cos(phi) * cos(psi) + sin(phi) * sin(theta) * sin(psi),...
       sin(phi) * cos(theta); sin(phi) * sin(psi)...
       + cos(phi) * sin(theta) * cos(psi), -sin(phi) * cos(psi)...
       + cos(phi) * sin(theta) * sin(psi), cos(phi) * cos(theta)];
          
  % Gravity, Thrust, Aerodynamic and Ground Forces
  W_FB = [-p.g * m * sin(theta), m * p.g * cos(theta) * sin(phi),...
            m * p.g * cos(theta) * cos(phi)]';
  T_FB = k(7: 9); FA_FB = k(1: 3); LG_FB = l(1: 3);
  F_FB = W_FB + T_FB + FA_FB + LG_FB; % total forces
      
  % Thrust, Aerodynamic and Ground Moments
  MT_FB = k(10: 12); MA_FB = k(4: 6); MLG_FB = l(4: 6);
  M_FB = MT_FB + MA_FB + MLG_FB; % total moments
  
  % Equations of Motion
  IBw = IB * x(4: 6);
  % Translational Dynamics  
  u_tran = F_FB ./ m - (mdot / p.m1) * x(1: 3) - cross(x(4: 6), x(1: 3));
  % Rotational Dynamics
  u_rot = IB \ M_FB - IB \ (cross(x(4: 6), IBw)) - IB \ IBdot * x(4: 6);
  % Translational Kinematics
  x_tran= B' * x(1: 3);
  % Rotational Kinematics
  x_rot = [x(4) + (x(5) * sin(phi) + x(6) * cos(phi)) * tan(theta),...
           x(5) * cos(phi) - x(6) * sin(phi),...
           (x(5) * sin(phi) + x(6) * cos(phi)) * sec(theta)]';
  
  xdot = [u_tran; u_rot; x_rot; x_tran];  % aircraft state variation with time
  
  % Immobilization
  if x(1) <= 1 && u(1) == 0 && x(12) >= href - 5
    xdot = [0 0 0 0 0 0 0 0 0 0 0 0]';
  end
  
end

== matlab function Model/Landing Gear Model/Landing Gear Model ==
  data: xdot input; y output; x input; href input; delta_bp input
function y  = LandingGear(xdot, x, href, delta_bp)

  z_corr = -(-x(12) + href);  % ground elevation corrected height
  xac = 1.9805;  % aerodynamic center position in x-axis
  phi = x(7);
  theta = x(8);
  d_main = 0.3;  % main tire diameter
  d_front = 0.19;  % front tire diameter
  
  % Vertical Force and Tire Deflection
  
  % First back wheel
  xw1 = 2.05 - xac;  % wheel position in x-axis
  yw1 = 1.6875;  % wheel position in y-axis
  cv1 = 1000;  % damping constant
  
  [Fv1, delta_g1, zw1] = Fv(x, xdot, z_corr, d_main, xw1, yw1, cv1);
  
  % Second back wheel
  xw2 = 2.05 - xac;
  yw2 = -1.6875;
  cv2 = 1000;
  
  [Fv2, delta_g2, zw2] = Fv(x, xdot, z_corr, d_main, xw2, yw2, cv2);
  
  % Front wheel
  xw3 = 1.01 - xac;
  yw3 = 0;
  cv3 = 100;
  
  [Fv3, delta_g3, zw3] = Fv(x, xdot, z_corr, d_front, xw3, yw3, cv3);
  
  %Propeller
  xprop = 2.968 - xac;  % propeller position in x-axis
  zprop = 0.404;  % propeller lowest point position in z-axis
  
  Fvprop = Fv_prop(x, z_corr, zprop, xprop);
    
  %Longitudinal Force
  delta_bpmax = 1;  % max brake pedal deflection
  mi_bmax = 0.2;  % max brake friction coeff
  mi_b = mi_bmax * delta_bp / delta_bpmax;  % brake friction coeff
  mi_roll = 0.02;  % rolling friction coeff
  mi = mi_b + mi_roll;  % total friction coeff
    
  Fm1 = mi * Fv1;
  Fm2 = mi * Fv2;
  Fm3 = mi_roll * Fv3;
  Fmprop = mi_roll * Fvprop;
  
  % Forces Translation to body axes
  Fx1 = -cos(theta) * Fm1 - sin(theta) * Fv1;
  Fx2 = -cos(theta) * Fm2 - sin(theta) * Fv2;
  Fx3 = -cos(theta) * Fm3 - sin(theta) * Fv3;
  Fxprop = -cos(theta) * Fmprop - sin(theta) * Fvprop;
    
  Fy1 = -sin(theta) * sin(phi) * Fm1 - cos(theta) * sin(phi) * Fv1;
  Fy2 = -sin(theta) * sin(phi) * Fm2 - cos(theta) * sin(phi) * Fv2;
  Fy3 = -sin(theta) * sin(phi) * Fm3 - cos(theta) * sin(phi) * Fv3;
  Fyprop = -sin(theta) * sin(phi) * Fmprop - cos(theta) * sin(phi) * Fvprop;
    
  Fz1 = -sin(theta) * cos(phi) * Fm1 - cos(theta) * cos(phi) * Fv1;
  Fz2 = -sin(theta) * cos(phi) * Fm2 - cos(theta) * cos(phi) * Fv2;
  Fz3 = -sin(theta) * cos(phi) * Fm3 - cos(theta) * cos(phi) * Fv3;
  Fzprop = -sin(theta) * cos(phi) * Fmprop - cos(theta) * cos(phi) * Fvprop;
  
  
  % Total forces
  X_LG = Fx1 + Fx2 + Fx3 + Fxprop;  
  Y_LG = Fy1 + Fy2 + Fy3 + Fyprop;
  Z_LG = Fz1 + Fz2 + Fz3 + Fzprop;
  
  % Rolling moment
  L1 = -(zw1 - delta_g1) * Fy1 + yw1 * Fz1;
  L2 = -(zw2 - delta_g2) * Fy2 + yw2 * Fz2;
  L3 = -(zw3 - delta_g3) * Fy3;
  Lprop = -zprop * Fyprop;
  
  % Pitching moment
  M1 = (zw1 - delta_g1) * Fx1 + xw1 * Fz1;
  M2 = (zw2 - delta_g2) * Fx2 + xw2 * Fz2;
  M3 = (zw3 - delta_g3) * Fx3 + xw3 * Fz3;
  Mprop = zprop * Fxprop + xprop * Fzprop;
  
  % Yawing moment
  N1 = -yw1 * Fx1 + xw1 * Fy1;
  N2 = -yw2 * Fx2 + xw2 * Fy2;
  N3 = xw3 * Fy3;
  Nprop = xprop * Fyprop;
  
  % Total moments
  L_LG = L1 + L2 + L3 + Lprop;
  M_LG = M1 + M2 + M3 + Mprop;
  N_LG = N1 + N2 + N3 + Nprop;

  y = [X_LG, Y_LG, Z_LG, L_LG, M_LG, N_LG]';
  
end
